simulink library "subPlatform_cl"  (R2018b)
settings: Solver=VariableStepAuto  StartTime=0.0  StopTime=10.0  RelTol=1e-3
values from neighbouring files (symbols this model uses):
  CB2CMVec = [0 0 0]    [simpSubPlatform_ts.m]
  flow = [0 0 0]    [simpSubPlatform_ts.m]
  grav = 9.81    [simpSubPlatform_ts.m]
  inertiaMatrix = eye(3)    [simpSubPlatform_ts.m]
  m = mass    (= 3333.33333333)    [simpSubPlatform_ts.m]
  tetherLengths = (norm(initPos+thr1Pt-thr1GndPos))*ones(3,1)    [simpSubPlatform_ts.m]
  thr1Pt = [0 1 -.5]    [simpSubPlatform_ts.m]
  thr2Pt = [cosd(30),-sind(30),-.5]    [simpSubPlatform_ts.m]
  thr3Pt = [-cosd(30),-sind(30),-.5]    [simpSubPlatform_ts.m]
  xOcean = 0    [simpSubPlatform_ts.m]
  xOceanPeriod = 10    [simpSubPlatform_ts.m]
  zOcean = -1000    [simpSubPlatform_ts.m]
  zOceanPeriod = 18    [simpSubPlatform_ts.m]
libraries: vrlib x4, eulAng2RotMat_ul x1, sixDoFDynamics_ul x1, tethers_cl x1, tethersMoment_cl x1, variableBuoyancy x1
settings Model: Creator=Erin B  LastModifiedBy=Erin B

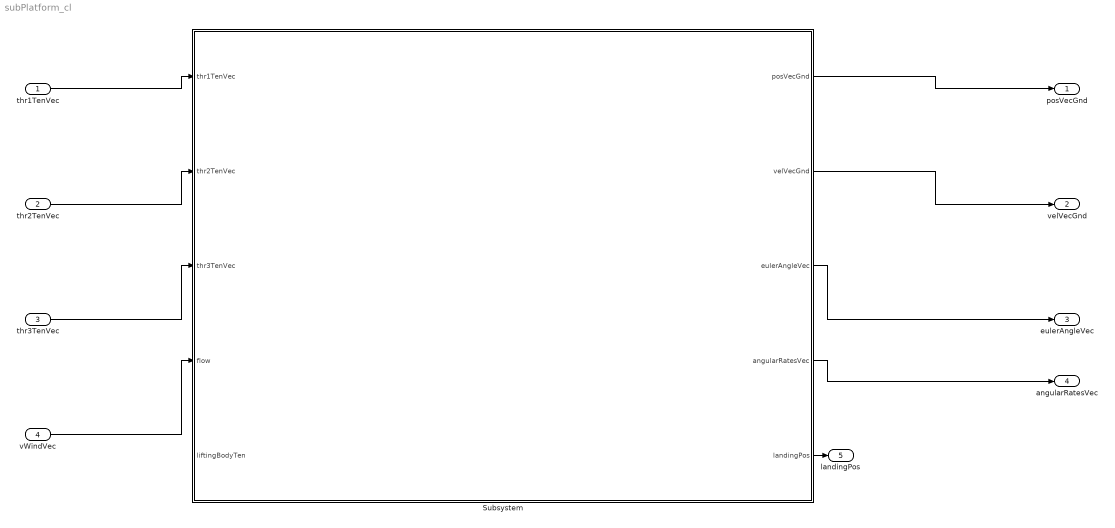
== system subPlatform_cl ==
  thr1TenVec : Inport
  thr2TenVec : Inport  Port=2
  thr3TenVec : Inport  Port=3
  vWindVec : Inport  Port=4
  Subsystem : Subsystem
  posVecGnd : Outport
  velVecGnd : Outport  Port=2
  eulerAngleVec : Outport  Port=3
  angularRatesVec : Outport  Port=4
  "landingPos " : Outport  Port=5
  wires:
  thr1TenVec/1 -> Subsystem/1(thr1TenVec)
  thr2TenVec/1 -> Subsystem/2(thr2TenVec)
  thr3TenVec/1 -> Subsystem/3(thr3TenVec)
  vWindVec/1 -> Subsystem/4(flow)
  Subsystem/1(posVecGnd) -> posVecGnd/1
  Subsystem/2(velVecGnd) -> velVecGnd/1
  Subsystem/3(eulerAngleVec) -> eulerAngleVec/1
  Subsystem/4(angularRatesVec) -> angularRatesVec/1
  Subsystem/5(landingPos) -> "landingPos "/1

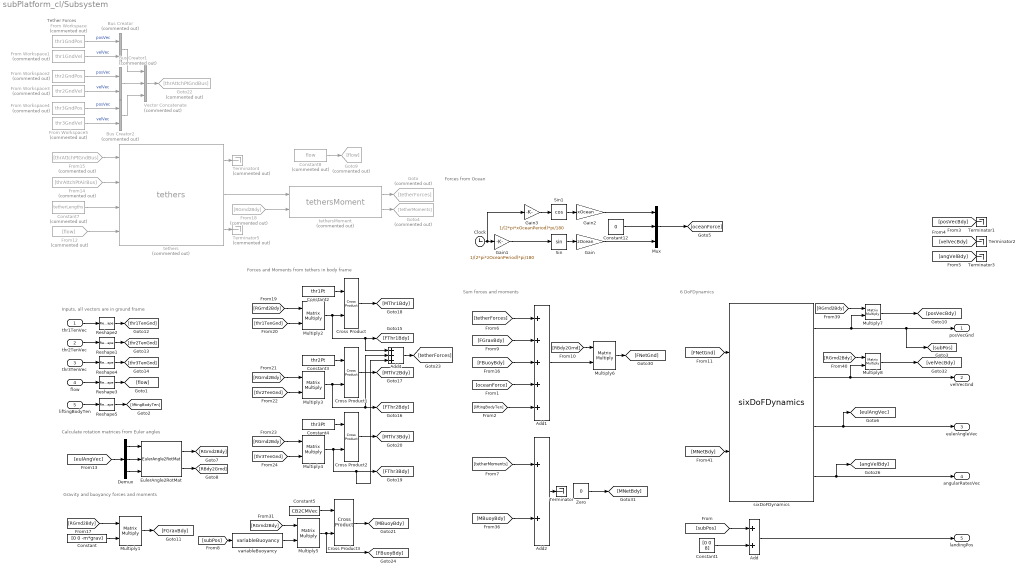
== system subPlatform_cl/Subsystem ==
  note: Tether Forces
  note: Inputs, all vectors are in ground frame
  note: Calculate rotation matrices from Euler angles
  note: Forces and Moments from tethers in body frame
  note: Sum forces and moments
  note: Gravity and buoyancy forces and moments
  note: 6 DoFDynamics
  note: Forces from Ocean
  thr1TenVec : Inport
  thr2TenVec : Inport  Port=2
  thr3TenVec : Inport  Port=3
  flow : Inport  Port=4
  liftingBodyTen : Inport  Port=5
  Add : Sum
  Add1 : Sum  Inputs=+++++
  Add2 : Sum
  Add4 : Sum  Inputs=+++
  Bus Creator : BusCreator  Commented=on  Inputs=2
  Bus Creator1 : BusCreator  Commented=on  Inputs=2
  Bus Creator2 : BusCreator  Commented=on  Inputs=2
  Clock : Clock
  Constant : Constant  Value=[0 0 -m*grav]
  Constant1 : Constant  Value=[0 0 8]
  Constant12 : Constant  Value=0
  Constant2 : Constant  Value=thr1Pt
  Constant3 : Constant  Value=thr2Pt
  Constant4 : Constant  Value=thr3Pt
  Constant5 : Constant  Value=CB2CMVec
  Constant7 : Constant  Commented=on  Value=tetherLengths
  Constant8 : Constant  Commented=on  Value=flow
  Cross Product{,1..3} (4 alike) : vrlib/Utilities/Cross Product
      settings: SourceProductBaseCode=VR
  Demux : Demux  Outputs=3
  EulerAngle2RotMat : eulAng2RotMat_ul/EulerAngle2RotMat  SystemSampleTime=-1
  From Workspace : FromWorkspace  Commented=on  VariableName=thr1GndPos  SampleTime=0
  From Workspace1 : FromWorkspace  Commented=on  VariableName=thr1GndVel  SampleTime=0
  From Workspace2 : FromWorkspace  Commented=on  VariableName=thr2GndPos  SampleTime=0
  From Workspace3 : FromWorkspace  Commented=on  VariableName=thr2GndVel  SampleTime=0
  From Workspace4 : FromWorkspace  Commented=on  VariableName=thr3GndPos  SampleTime=0
  From Workspace5 : FromWorkspace  Commented=on  VariableName=thr3GndVel  SampleTime=0
  From12 : From  Commented=on  GotoTag=flow
  From14 : From  Commented=on  GotoTag=thrAttchPtAirBus
  From15 : From  Commented=on  GotoTag=thrAttchPtGndBus
  From18 : From  Commented=on  GotoTag=RGrnd2Bdy
  Gain : Gain  Gain=zOcean
  Gain1 : Gain  Gain=1/(2*pi*zOceanPeriod)*pi/180
  Gain2 : Gain  Gain=xOcean
  Gain3 : Gain  Gain=1/(2*pi*xOceanPeriod)*pi/180
  Goto : Goto  Commented=on  GotoTag=tetherForces
  Goto22 : Goto  Commented=on  GotoTag=thrAttchPtGndBus
  Goto4 : Goto  Commented=on  GotoTag=tetherMoments
  Goto9 : Goto  Commented=on  GotoTag=flow
  Multiply{1..8} (8 alike) : Product  Multiplication=Matrix(*)
  Mux : Mux  Inputs=3
  Reshape{1..5} (5 alike) : Reshape  OutputDimensionality=Column vector (2-D)
  Sin : Trigonometry  OutputSignalType=real
  Sin1 : Trigonometry  Operator=cos  OutputSignalType=real
  Terminator{,1..3} (4 alike) : Terminator
  Terminator4 : Terminator  Commented=on
  Terminator5 : Terminator  Commented=on
  Vector Concatenate : Concatenate  Commented=on  NumInputs=3
  Zero : Constant  Value=0  OutDataTypeStr=Inherit: Inherit via back propagation
  sixDoFDynamics : sixDoFDynamics_ul/sixDoFDynamics  M=mass  initPos=initPos  initVel=initVel  J=inertiaMatrix  initEulAngs=initEulerAngles  initAngVel=initAngVel
  tethers : tethers_cl/tethers  Commented=on  thr=thr
  tethersMoment : tethersMoment_cl/tethersMoment  Commented=on  arms=arms
  variableBuoyancy : variableBuoyancy/variableBuoyancy  vol=vol  h=h  grav=grav  rho=rho  waveAmplitude=waveAmp  oceanDepth=oceanDepth  wavePeriod=wavePeriod
  posVecGnd : Outport
  velVecGnd : Outport  Port=2
  eulerAngleVec : Outport  Port=3
  angularRatesVec : Outport  Port=4
  landingPos : Outport  Port=5
  wires:
  [RBdy2Grnd] -> Multiply6/1
  Add2/1 -> Terminator/1
  flow/1 -> Reshape3/1
  EulerAngle2RotMat/2 -> [RBdy2Grnd]
  Multiply4/1 -> Add4/3, [FThr3Bdy], Cross Product2/2
  sixDoFDynamics/4 -> angularRatesVec/1, [angVelBdy]
  variableBuoyancy/1 -> Multiply5/2
  Constant3/1 -> Cross Product1/1
  Multiply8/1 -> [velVecBdy]
  Cross Product/1 -> [MThr1Bdy]
  [thr2TenGnd] -> Multiply3/2
  [MBuoyBdy] -> Add2/2
  Reshape2/1 -> [thr1TenGnd]
  liftingBodyTen/1 -> Reshape5/1
  [tetherMoments] -> Add2/1
  [liftingBodyTen] -> Add1/5
  [thr3TenGnd] -> Multiply4/2
  [FGravBdy] -> Add1/2
  Zero/1 -> [MNetBdy]
  [FBuoyBdy] -> Add1/3
  [oceanForce] -> Add1/4
  tethersMoment/1 -> Goto/1
  tethersMoment/2 -> Goto4/1
  thr2TenVec/1 -> Reshape1/1
  [FNetGnd] -> sixDoFDynamics/1
  tethers/3 -> Terminator5/1
  thr3TenVec/1 -> Reshape4/1
  Cross Product2/1 -> [MThr3Bdy]
  From15/1 -> tethers/1
  Add1/1 -> Multiply6/2
  Cross Product1/1 -> [MThr2Bdy]
  Demux/2 -> EulerAngle2RotMat/2
  sixDoFDynamics/2 -> velVecGnd/1, Multiply8/2
  From12/1 -> tethers/4
  [RGrnd2Bdy] -> Multiply5/1
  [subPos] -> Add/1
  Add/1 -> landingPos/1
  Multiply7/1 -> [posVecBdy]
  tethers/2 -> tethersMoment/1
  Cross Product3/1 -> [MBuoyBdy]
  tethers/1 -> Terminator4/1
  [RGrnd2Bdy] -> Multiply3/1
  sixDoFDynamics/3 -> eulerAngleVec/1, [eulAngVec]
  Multiply1/1 -> [FGravBdy]
  Multiply5/1 -> Cross Product3/2, [FBuoyBdy]
  Constant/1 -> Multiply1/2
  From14/1 -> tethers/2
  sixDoFDynamics/1 -> [subPos], posVecGnd/1, Multiply7/2
  Reshape5/1 -> [liftingBodyTen]
  Multiply6/1 -> [FNetGnd]
  Constant4/1 -> Cross Product2/1
  From18/1 -> tethersMoment/2
  [RGrnd2Bdy] -> Multiply4/1
  Reshape1/1 -> [thr2TenGnd]
  Demux/1 -> EulerAngle2RotMat/1
  Constant5/1 -> Cross Product3/1
  [RGrnd2Bdy] -> Multiply2/1
  thr1TenVec/1 -> Reshape2/1
  [eulAngVec] -> Demux/1
  Demux/3 -> EulerAngle2RotMat/3
  [RGrnd2Bdy] -> Multiply1/1
  [RGrnd2Bdy] -> Multiply8/1
  [RGrnd2Bdy] -> Multiply7/1
  Multiply2/1 -> Add4/1, [FThr1Bdy], Cross Product/2
  Reshape3/1 -> [flow]
  [thr1TenGnd] -> Multiply2/2
  [tetherForces] -> Add1/1
  EulerAngle2RotMat/1 -> [RGrnd2Bdy]
  Constant2/1 -> Cross Product/1
  Multiply3/1 -> Add4/2, [FThr2Bdy], Cross Product1/2
  Reshape4/1 -> [thr3TenGnd]
  Constant7/1 -> tethers/3
  [MNetBdy] -> sixDoFDynamics/2
  Constant1/1 -> Add/2
  Sin/1 -> Gain/1
  Constant12/1 -> Mux/2
  Gain2/1 -> Mux/1
  Gain1/1 -> Sin/1
  Mux/1 -> [oceanForce]
  Gain/1 -> Mux/3
  Gain3/1 -> Sin1/1
  Clock/1 -> Gain3/1, Gain1/1
  Sin1/1 -> Gain2/1
  Constant8/1 -> Goto9/1
  From Workspace/1 -> Bus Creator/1  "posVec"
  From Workspace1/1 -> Bus Creator/2  "velVec"
  Bus Creator/1 -> Vector Concatenate/1
  From Workspace3/1 -> Bus Creator1/2  "velVec"
  Bus Creator1/1 -> Vector Concatenate/2
  From Workspace2/1 -> Bus Creator1/1  "posVec"
  From Workspace5/1 -> Bus Creator2/2  "velVec"
  Bus Creator2/1 -> Vector Concatenate/3
  From Workspace4/1 -> Bus Creator2/1  "posVec"
  Vector Concatenate/1 -> Goto22/1
  Add4/1 -> [tetherForces]
  [subPos] -> variableBuoyancy/1
